simulink model "model1"  (R2017a)
settings: Solver=VariableStepAuto  StartTime=0.0  StopTime=30  RelTol=1e-9
values from neighbouring files (symbols this model uses):
  K = 0.9    [main.m]
  R = r0*[1 -1]    [main.m]
  S = [(z0^2+As(2)*r0)/Bs (-2*z0-(As(2)-1))/Bs]    [main.m]
  T = [t1 t0]    [main.m]
  taux = tr_BO/3    (= 0.1)    [main.m]
  Ts = 30*1e-3    (= 0.03)    [main.m]
settings Model: Creator=GANOU Arouna  LastModifiedBy=GANOU Arouna

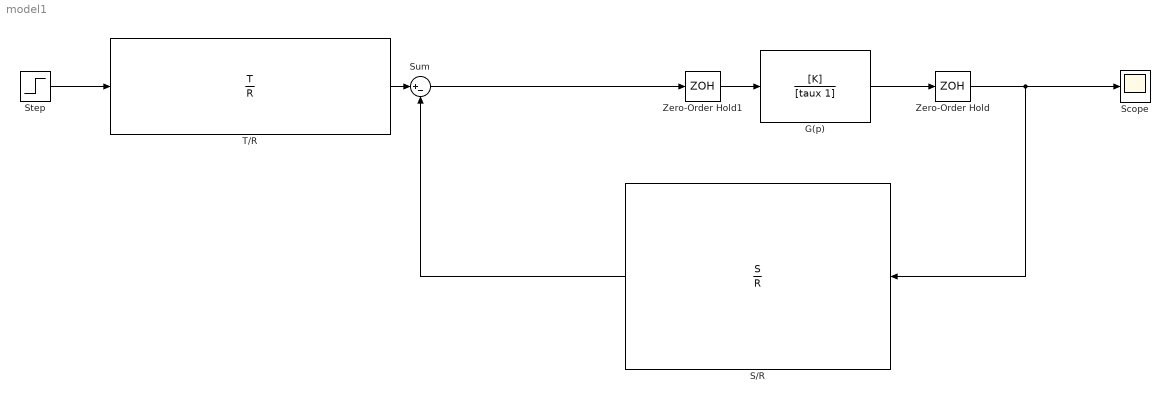
== system model1 ==
  G(p) : TransferFcn  Numerator=[K]  Denominator=[taux 1]
  S/R : DiscreteTransferFcn  Numerator=S  Denominator=R  SampleTime=Ts
  Scope : Scope
  Step : Step  After=5  SampleTime=Ts
  Sum : Sum  Inputs=|+-
  T/R : DiscreteTransferFcn  Numerator=T  Denominator=R  SampleTime=Ts
  Zero-Order Hold : ZeroOrderHold  SampleTime=Ts
  Zero-Order Hold1 : ZeroOrderHold  SampleTime=Ts
  wires:
  Step/1 -> T/R/1
  T/R/1 -> Sum/1
  Sum/1 -> Zero-Order Hold1/1
  Zero-Order Hold1/1 -> G(p)/1
  G(p)/1 -> Zero-Order Hold/1
  Zero-Order Hold/1 -> S/R/1, Scope/1
  S/R/1 -> Sum/2
